simulink model "sensorExpolerFORPROTEN (2)"  (R2026a)
settings: Solver=FixedStepDiscrete  StopTime=inf  FixedStep=0.001
undefined symbols (not defined in the file): Blocking, Non
libraries: amg_usbconverter_n_connect_lib x2
settings Model: Creator=pboon  LastModifiedBy=focus

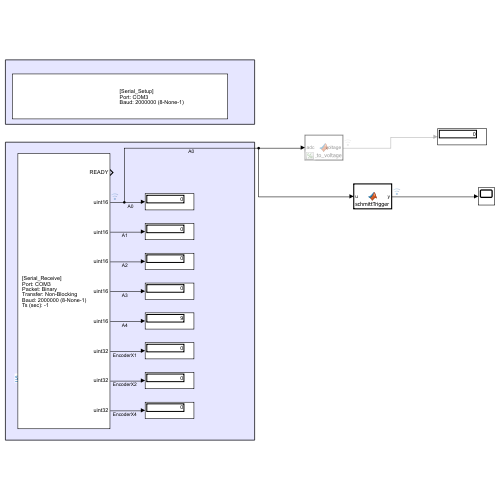
[thumbnail: Simulink's stored preview of the top-level diagram]
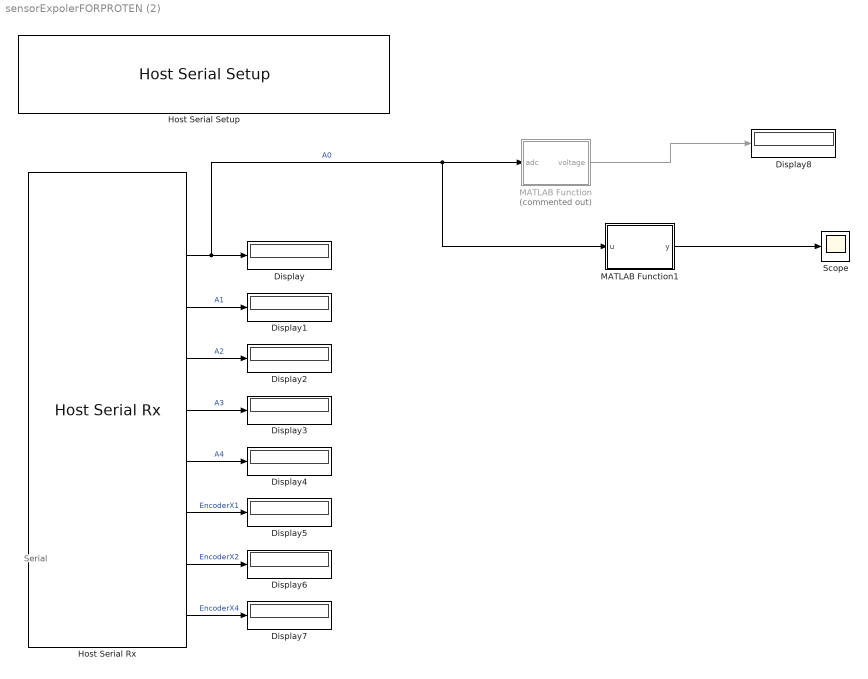
== system sensorExpolerFORPROTEN (2) ==
  note: Serial
  Display{,1..8} (9 alike) : Display
  Host Serial Rx : amg_usbconverter_n_connect_lib/Host Serial Rx  conf=rx  port=<auto>  baudrate=2000000  databits=8  parity=None  stopbit=1  flowcontrol=None  transfer=Non-Blocking  timeout=5  packetmode=Binary  enableinitialvalues=off  initialvalues=[]  binheader='25'  binterminator='4E 4E'  porttype_double=0  porttype_single=0  porttype_int8=0  porttype_uint8=0  porttype_int16=0  porttype_uint16=5  porttype_int32=0  porttype_uint32=3  asciiformat='%d,%f'  rx_asciiterminator="CRLF (0x0D 0x0A - \"\\r\\n\")"  tx_asciiterminator="CRLF (0x0D 0x0A - \"\\r\\n\")"  sampletime=0.001  enablecustomportlabel=off  cinputportlabel=0  coutputportlabel=A  portpinstr=0  blockid=HostSerialRx  inputporttype=[]  inputportwidth=[]  inputportlabel={}  outputporttype=[3 5 5 5 5 5 7 7 7]  outputportwidth=[1 1 1 1 1 1 1 1 1]  outputportlabel={'READY','uint16','uint16','uint16','uint16','uint16','uint32','uint32','uint32'}  compat=0  optionstring=[]  autoport='COM3'
  Host Serial Setup : amg_usbconverter_n_connect_lib/Host Serial Setup  conf=setup  port=<auto>  baudrate=2000000  databits=8  parity=None  stopbit=1  flowcontrol=None  transfer=Blocking  timeout=2  packetmode=Binary  initialvalues=[]  binheader='7E 7E'  binterminator='03 03'  porttype_double=0  porttype_single=1  porttype_int8=0  porttype_uint8=0  porttype_int16=0  porttype_uint16=0  porttype_int32=0  porttype_uint32=2  asciiformat='%d %u %x'  rx_asciiterminator="CRLF (0x0D 0x0A - \"\\r\\n\")"  tx_asciiterminator="CRLF (0x0D 0x0A - \"\\r\\n\")"  sampletime=-1  enablecustomportlabel=off  cinputportlabel=0  coutputportlabel=A  portpinstr=0  blockid=HostSerialSetup  inputporttype=[]  inputportwidth=[]  inputportlabel={}  outputporttype=[]  outputportwidth=[]  outputportlabel={}  compat=0  optionstring=[]  autoport='COM3'
  MATLAB Function : MATLAB Function  Commented=on  TreatAsAtomicUnit=on
  MATLAB Function1 : MATLAB Function  TreatAsAtomicUnit=on
  Scope : Scope
      settings: ActiveDisplayYMinimum=-1  ActiveDisplayYMaximum=1
  wires:
  Host Serial Rx/2 -> MATLAB Function1/1(u), MATLAB Function/1(adc), Display/1  "A0"
  Host Serial Rx/3 -> Display1/1  "A1"
  Host Serial Rx/4 -> Display2/1  "A2"
  Host Serial Rx/5 -> Display3/1  "A3"
  Host Serial Rx/6 -> Display4/1  "A4"
  Host Serial Rx/7 -> Display5/1  "EncoderX1"
  Host Serial Rx/8 -> Display6/1  "EncoderX2"
  Host Serial Rx/9 -> Display7/1  "EncoderX4"
  MATLAB Function/1(voltage) -> Display8/1
  MATLAB Function1/1(y) -> Scope/1

== matlab function sensorExpolerFORPROTEN (2)/MATLAB Function ==
  data: adc input; voltage output
function voltage = adc_to_voltage(adc)
%#codegen
Vref = 3.3;
voltage = (double(adc) / 4095) * Vref;
end

== matlab function sensorExpolerFORPROTEN (2)/MATLAB Function1 ==
  data: u input; y output
function y = schmittTrigger(u)
%#codegen
% Schmitt Trigger รับ ADC เพียง 1 ช่อง (เช่น A0 จาก Potentiometer)
% แปลงเป็น Digital Output 0/1 แบบมี Hysteresis

    UT = uint16(2200);   % Upper Threshold (ปรับตามค่าจริงที่วัดได้)
    LT = uint16(1800);   % Lower Threshold

    persistent state
    if isempty(state)
        state = uint8(0);   % เริ่มต้นที่ 0
    end

    if u > UT
        state = uint8(1);
    elseif u < LT
        state = uint8(0);
    end
    % ถ้าอยู่ระหว่าง LT-UT: คงค่าเดิม (Hysteresis)

    y = state;
end
